simulink model "SimulinkTP1"  (R2018b)
settings: Solver=VariableStepAuto  StartTime=0.0  StopTime=0.0025  RelTol=1e-3
libraries: fl_lib x7, nesl_utility x4
settings Model: Creator=A47521  LastModifiedBy=A47521
settings DebuggingCC: UnconnectedInputMsg=none  UnconnectedOutputMsg=none  UnconnectedLineMsg=none

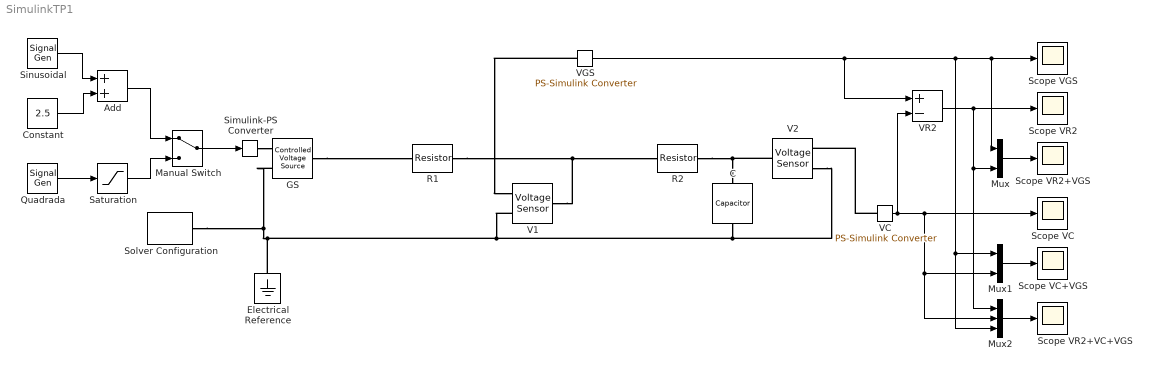
== system SimulinkTP1 ==
  Add : Sum
  C : fl_lib/Electrical/Electrical Elements/Capacitor  c=100 nF  r=1e-6 Ohm  g=0 1/Ohm  i_specify=off  i_priority=None  i=0 A  i_nominal_specify=off  i_nominal_unit=A  i_nominal_value=1  v_specify=off  v_priority=None  v=0 V  v_nominal_specify=off  v_nominal_unit=V  v_nominal_value=1  vc_specify=off  vc_priority=High  vc=0 V  vc_nominal_specify=off  vc_nominal_unit=V  vc_nominal_value=1
  Constant : Constant  Value=2.5
  Electrical Reference : fl_lib/Electrical/Electrical Elements/Electrical Reference
  GS : fl_lib/Electrical/Electrical Sources/Controlled Voltage Source
  Manual Switch : ManualSwitch
  Mux : Mux  Inputs=2
  Mux1 : Mux  Inputs=2
  Mux2 : Mux  Inputs=3
  Quadrada : SignalGenerator  WaveForm=square  Amplitude=5  Frequency=1000
  R1 : fl_lib/Electrical/Electrical Elements/Resistor  R=50 Ohm  i_specify=off  i_priority=None  i=0 A  i_nominal_specify=off  i_nominal_unit=A  i_nominal_value=1  v_specify=off  v_priority=None  v=0 V  v_nominal_specify=off  v_nominal_unit=V  v_nominal_value=1
  R2 : fl_lib/Electrical/Electrical Elements/Resistor  R=2.2 kOhm  i_specify=off  i_priority=None  i=0 A  i_nominal_specify=off  i_nominal_unit=A  i_nominal_value=1  v_specify=off  v_priority=None  v=0 V  v_nominal_specify=off  v_nominal_unit=V  v_nominal_value=1
  Saturation : Saturate  UpperLimit=5  LowerLimit=0
  Scope VC : Scope
  Scope VC+VGS : Scope
  Scope VGS : Scope
  Scope VR2 : Scope
  Scope VR2+VC+VGS : Scope
  Scope VR2+VGS : Scope
  Simulink-PS Converter : nesl_utility/Simulink-PS Converter  PhysicalDomain=network_engine_domain  SubClassName=ps_input  LeftPortType=input  RightPortType=output  PseudoPeriodic=off  Frequencies=[]  NoiseDistribution=none  NoiseParameters=[]  Unit=1  AffineConversion=off  FilteringAndDerivatives=provide  SimscapeFilterOrder=1  InputFilterTimeConstant=0.001  UdotUserProvided=0
  Sinusoidal : SignalGenerator  Amplitude=2.5  Frequency=1000
  Solver Configuration : nesl_utility/Solver Configuration  PhysicalDomain=network_engine_domain  SubClassName=solver  LeftPortType=input  RightPortType=generic  Tones=[]  Harmonics=[]  SimulateNoise=off  Profile=off  UseLocalSampling=off  EnableSwitchedLinearOptims=on  FrequencyDomain=off  UseCCode=off  RelTol=0.001  AbsTol=1e-06  MinStep=1e-09  ToWorkspace=off  RevertToSquareIcSolve=off  NumHomotopyIterations=100  PhasorMode=off  PhasorModeNumHarmonics=1  DoDC=off  ResidualTolerance=1e-09  UseLocalSolver=off  LocalSolverChoice=NE_BACKWARD_EULER_ADVANCER  LocalSolverSampleTime=0.001  DoFixedCost=off  MaxNonlinIter=3  MaxModeIter=2  LinearAlgebra=auto  EquationFormulation=NE_TIME_EF  DelaysMemoryBudget=1024  AutomaticFiltering=on  FilteringTimeConstant=0.001  PartitionStorageMethod=AS_NEEDED  PartitionMemoryBudget=1024
  V1 : fl_lib/Electrical/Electrical Sensors/Voltage Sensor
  V2 : fl_lib/Electrical/Electrical Sensors/Voltage Sensor
  VC : nesl_utility/PS-Simulink Converter  PhysicalDomain=network_engine_domain  SubClassName=ps_output  LeftPortType=input  RightPortType=output  PseudoPeriodic=off  Frequencies=[]  Unit=1  AffineConversion=off
  VGS : nesl_utility/PS-Simulink Converter  PhysicalDomain=network_engine_domain  SubClassName=ps_output  LeftPortType=input  RightPortType=output  PseudoPeriodic=off  Frequencies=[]  Unit=1  AffineConversion=off
  VR2 : Sum  Inputs=+-
  wires:
  VGS/1 -> VR2/1, Mux2/3, Mux1/1, Mux/1, Scope VGS/1
  Mux/1 -> Scope VR2+VGS/1
  VC/1 -> VR2/2, Scope VC/1, Mux2/2, Mux1/2
  Quadrada/1 -> Saturation/1
  Mux1/1 -> Scope VC+VGS/1
  VR2/1 -> Mux/2, Mux2/1, Scope VR2/1
  Sinusoidal/1 -> Add/1
  Constant/1 -> Add/2
  Mux2/1 -> Scope VR2+VC+VGS/1
  Manual Switch/1 -> Simulink-PS Converter/1
  Saturation/1 -> Manual Switch/2
  Add/1 -> Manual Switch/1
  connections:
  Electrical Reference/LConn1 -- V2/RConn2 -- C/RConn1 -- V1/RConn2 -- GS/RConn2 -- Solver Configuration/RConn1
  VGS/LConn1 -- V1/RConn1
  VC/LConn1 -- V2/RConn1
  Simulink-PS Converter/RConn1 -- GS/RConn1
  GS/LConn1 -- R1/LConn1
  R1/RConn1 -- V1/LConn1 -- R2/LConn1
  R2/RConn1 -- C/LConn1 -- V2/LConn1
